simulink model "Q1_PI_controller"  (R2017a)
settings: Solver=FixedStepDiscrete  StartTime=0.0  StopTime=15  FixedStep=5e-5  RelTol=1e-3
libraries: powerlib x5, electricdrivelib x1, peDiscretePi x1
settings Model: Creator=nailt  LastModifiedBy=nailt

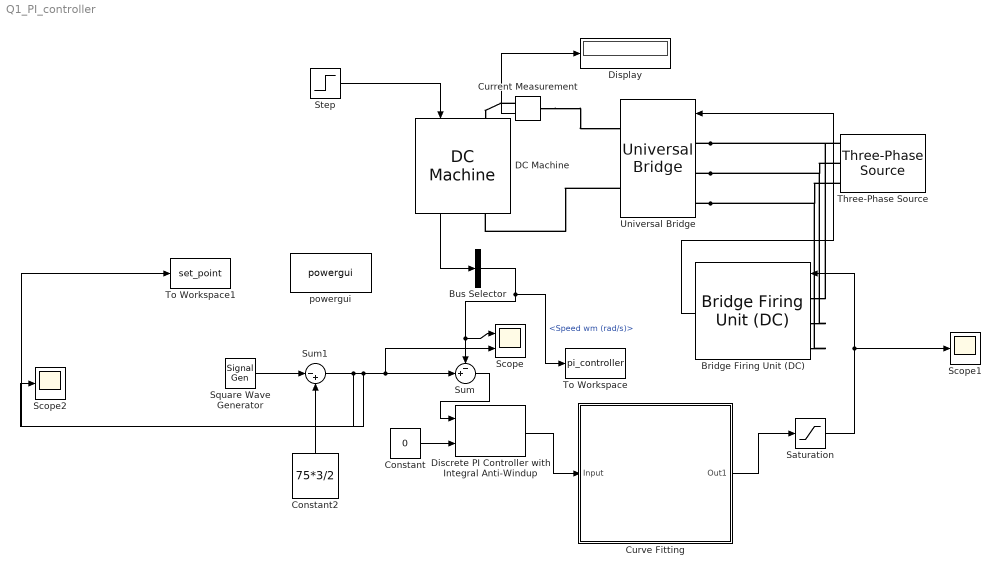
== system Q1_PI_controller ==
  Bridge Firing Unit (DC) : electricdrivelib/Fundamental Drive Blocks/Bridge Firing Unit (DC)  OverrideUsingVariant=AC_Detailed_two quadrant  detailLevel=Detailed  nbPhases=3  numQuad=2  x4=50  x9=10  Ts=50e-6
      settings: SourceProductName=Simscape Power Systems  SourceProductBaseCode=PS
  Bus Selector : BusSelector  OutputSignals=Speed wm (rad/s)
  Constant : Constant  Value=0
  Constant2 : Constant  Value=75*3/2
  Current Measurement : powerlib/Measurements/Current Measurement  PhasorSimulation=off  OutputType=Complex  PSBequivalent=0
  Curve Fitting : Subsystem
  DC Machine : powerlib/Machines/DC Machine  PresetModel=No  MechanicalLoad=Torque TL  FieldType=Permanent magnet  ShowDetailedParameters=on  MeasurementBus=off  RLa=[10 0.1]  RLf=[281.3 156]  Laf=0.9483  MachineConstant=Back-emf constant (V/rpm)  Ke=0.3  Kt=1.8  J=0.4  Bm=0.002953  Tf=0.5161  w0=1  Ifinit=1  TsPowergui=0  TsBlock=-1
  Discrete PI Controller with Integral Anti-Windup : peDiscretePi/Discrete PI Controller with Integral Anti-Windup  Kp=25  Ki=25  x0=0  B=150  A=0  Ts=1/50
  Display : Display
  Saturation : Saturate  UpperLimit=150  LowerLimit=0.00001
  Scope : Scope  NumInputPorts=2
  Scope1 : Scope
  Scope2 : Scope
  Square Wave Generator : SignalGenerator  WaveForm=square  Amplitude=75/2  Frequency=1/9
  Step : Step  Time=0.001  After=24  SampleTime=5e-5
  Sum : Sum  Inputs=-+|
  Sum1 : Sum  Inputs=|-+
  Three-Phase Source : powerlib/Electrical Sources/Three-Phase Source  InternalConnection=Yg  VoltagePhases=off  Voltage=400  PhaseAngle=0  Voltage_phases=[25e3 25e3 25e3]/sqrt(3)  PhaseAngles_phases=[0 -120 +120]  Frequency=50  NonIdealSource=on  SpecifyImpedance=off  Resistance=100e-3  Inductance=100e-6  ShortCircuitLevel=100e6  BaseVoltage=25e3  XRratio=7  BusType=swing  Pref=10e3  Qref=0  Prefabc=[10e3, 10e3, 10e3]  Qrefabc=[0, 0, 0]  Qmin=-inf  Qmax=inf
  To Workspace : ToWorkspace  VariableName=pi_controller  SaveFormat=Timeseries  SampleTime=-1
  To Workspace1 : ToWorkspace  VariableName=set_point  SaveFormat=Timeseries  SampleTime=-1
  Universal Bridge : powerlib/Power Electronics/Universal Bridge  Arms=3  SnubberResistance=1e10  SnubberCapacitance=inf  Device=Thyristors  Ron=20e-3  Lon=0  ForwardVoltages="[  0  0  ]"  ForwardVoltage=0.8  GTOparameters=[ 10e-6 , 20e-6 ]  IGBTparameters=[ 1e-6 , 2e-6 ]  Measurements=None  Measurements_2=None  converterType=Rectifier
  powergui : powerlib/powergui  Priority=1  SimulationMode=Discrete  SampleTime=50e-6  frequency=60  Iterations=50  frequencyindice=50  Pbase=100e6  ErrMax=1e-4  UnitsV=kV  UnitsW=MW  buscounter=0  FunctionMessages=off  echomessages=off  EnableUseOfTLC=off  CurrentSourceSwitches=off  DisableSnubberDevices=off  DisableRonSwitches=off  DisableVfSwitches=off  DisplayEquations=off  SolverType=Tustin/Backward Euler (TBE)  Interpol=off  ExternalGateDelay=off  methode=off  Ts=100  x0status=blocks  SPID=off  SwTol=0  HookPort=off  RestoreLinks=warning  ResistiveCurrentMeasurement=off  Frange=[0:2:500]  Ylog=off  Xlog=on  ShowGrid=off  save=off  variable=ZData  structure=0  ZoomFFT=off  StartTime=0.0  cycles=1  DisplayStyle=1  fundamental=60  FreqAxis=off  MaxFrequency=1000  frequencyindicesteady=1  RmsSteady=1  display=off
  wires:
  Sum/1 -> Discrete PI Controller with Integral Anti-Windup/1
  Bus Selector/1 -> To Workspace/1, Scope/1, Sum/1  "<Speed wm (rad/s)>"
  Step/1 -> DC Machine/1
  Current Measurement/1 -> Display/1
  Bridge Firing Unit (DC)/1 -> Universal Bridge/1
  Sum1/1 -> Scope2/1, To Workspace1/1, Scope/2, Sum/2
  DC Machine/1 -> Bus Selector/1
  Curve Fitting/1(Out1) -> Saturation/1
  Discrete PI Controller with Integral Anti-Windup/1 -> Curve Fitting/1(Input)
  Saturation/1 -> Scope1/1, Bridge Firing Unit (DC)/1
  Constant/1 -> Discrete PI Controller with Integral Anti-Windup/2
  Constant2/1 -> Sum1/2
  Square Wave Generator/1 -> Sum1/1
  connections:
  Universal Bridge/LConn3 -- Three-Phase Source/RConn3 -- Bridge Firing Unit (DC)/LConn3
  Universal Bridge/LConn2 -- Three-Phase Source/RConn2 -- Bridge Firing Unit (DC)/LConn2
  Universal Bridge/LConn1 -- Three-Phase Source/RConn1 -- Bridge Firing Unit (DC)/LConn1
  Current Measurement/RConn1 -- DC Machine/LConn1
  Universal Bridge/RConn2 -- DC Machine/RConn1
  Current Measurement/LConn1 -- Universal Bridge/RConn1

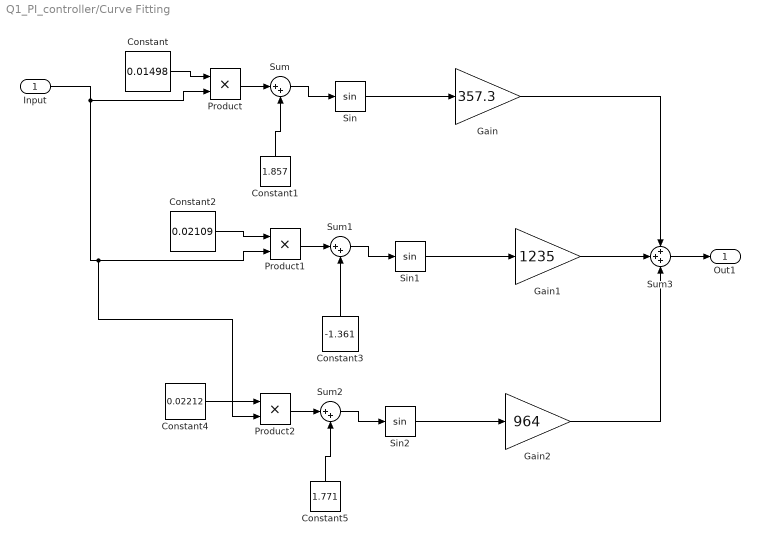
== system Q1_PI_controller/Curve Fitting ==
  Input : Inport
  Constant : Constant  Value=0.01498  SampleTime=5e-5
  Constant1 : Constant  Value=1.857
  Constant2 : Constant  Value=0.02109  SampleTime=5e-5
  Constant3 : Constant  Value=-1.361  SampleTime=5e-5
  Constant4 : Constant  Value=0.02212  SampleTime=5e-5
  Constant5 : Constant  Value=1.771  SampleTime=5e-5
  Gain : Gain  Gain=357.3
  Gain1 : Gain  Gain=1235
  Gain2 : Gain  Gain=964
  Product : Product
  Product1 : Product
  Product2 : Product
  Sin : Trigonometry
  Sin1 : Trigonometry
  Sin2 : Trigonometry
  Sum : Sum  Inputs=|++
  Sum1 : Sum  Inputs=|++
  Sum2 : Sum  Inputs=|++
  Sum3 : Sum  Inputs=3
  Out1 : Outport
  wires:
  Input/1 -> Product2/2, Product1/2, Product/2
  Sin2/1 -> Gain2/1
  Sin/1 -> Gain/1
  Constant/1 -> Product/1
  Sin1/1 -> Gain1/1
  Gain1/1 -> Sum3/2
  Product/1 -> Sum/1
  Sum/1 -> Sin/1
  Sum1/1 -> Sin1/1
  Sum2/1 -> Sin2/1
  Constant1/1 -> Sum/2
  Gain2/1 -> Sum3/3
  Constant4/1 -> Product2/1
  Constant5/1 -> Sum2/2
  Product2/1 -> Sum2/1
  Product1/1 -> Sum1/1
  Constant3/1 -> Sum1/2
  Gain/1 -> Sum3/1
  Constant2/1 -> Product1/1
  Sum3/1 -> Out1/1
